simulink model "model_2"  (R2021b)
settings: Solver=FixedStepAuto  StartTime=0.0  StopTime=3  FixedStep=0.00005  RelTol=1e-3
values from neighbouring files (symbols this model uses):
  A = [-6, 0, 0, 0; 0, 8,  0, 0; 0, 0, 2, 5; 0, 0, -5, 2]    [task_1.m]    (also in task_2.m = [0, 7, 0, 0; -7, 0,  0, 0; 0, 0, 0, 1; 0, 0, -1, 0]; task_3.m = [5, -9, -7, 1; -9, 5,  -1, 7; -7, -1, 5, 9; 1, 7, 9, 5])
  B = [0; 1; 9; 2]    [task_1.m]    (also in task_2.m = [0; 0; 0; 0]; task_3.m = [3; 3; 1; 3])
  C = [1, 0, 0, 0; 0, 1, 0, 0; 0, 0, 1, 0; 0, 0, 0, 1]    [task_1.m]    (also in task_2.m = [0, 5, 5, 0]; task_3.m = [2, -2, 2, 2; -2, 4, 2, 4])
  L = inv(Q) * Y    [task_2.m]    (also in task_3.m = inv(Q) * Y1)
  x0 = [1; 1; 1; 1]    [task_2.m]    (also in task_3.m)
  x_0 = [1; 1; 1; 1]    [task_1.m]    (also in task_2.m = [2; 0; 0; -1]; task_3.m = [2; 3; 4; -5])
settings Model: Creator=den  LastModifiedBy=vital

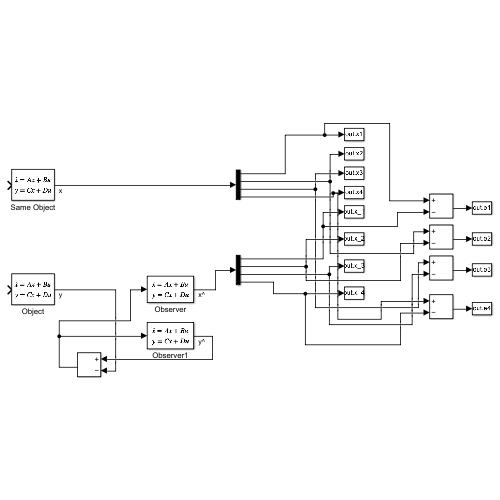
[thumbnail: Simulink's stored preview of the top-level diagram]
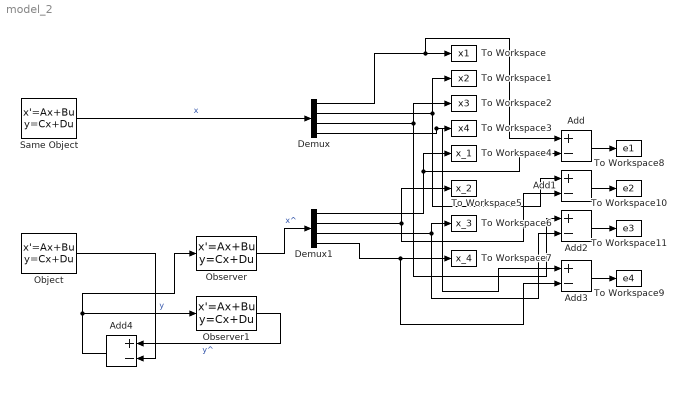
== system model_2 ==
  Add{,1..4} (5 alike) : Sum  Inputs=+-
  Demux : Demux
  Demux1 : Demux
  Object : StateSpace  A=A  B=B  C=C  D=0  InitialCondition=x0
  Observer : StateSpace  A=A  B=L  C=[1,0,0,0; 0,1,0,0; 0,0,1,0; 0,0,0,1]  D=[0;0;0;0]  InitialCondition=x_0  ParameterTunability=Unconstrained
  Observer1 : StateSpace  A=A  B=L  C=C  D=0  InitialCondition=x_0  ParameterTunability=Unconstrained
  Same Object : StateSpace  A=A  B=B  C=[1,0,0,0; 0,1,0,0; 0,0,1,0; 0,0,0,1]  D=[0; 0; 0; 0]  InitialCondition=x0  ParameterTunability=Unconstrained
  To Workspace : ToWorkspace  VariableName=x1  SaveFormat=Timeseries  SampleTime=-1
  To Workspace1 : ToWorkspace  VariableName=x2  SaveFormat=Timeseries  SampleTime=-1
  To Workspace10 : ToWorkspace  VariableName=e2  SaveFormat=Timeseries  SampleTime=-1
  To Workspace11 : ToWorkspace  VariableName=e3  SaveFormat=Timeseries  SampleTime=-1
  To Workspace2 : ToWorkspace  VariableName=x3  SaveFormat=Timeseries  SampleTime=-1
  To Workspace3 : ToWorkspace  VariableName=x4  SaveFormat=Timeseries  SampleTime=-1
  To Workspace4 : ToWorkspace  VariableName=x_1  SaveFormat=Timeseries  SampleTime=-1
  To Workspace5 : ToWorkspace  VariableName=x_2  SaveFormat=Timeseries  SampleTime=-1
  To Workspace6 : ToWorkspace  VariableName=x_3  SaveFormat=Timeseries  SampleTime=-1
  To Workspace7 : ToWorkspace  VariableName=x_4  SaveFormat=Timeseries  SampleTime=-1
  To Workspace8 : ToWorkspace  VariableName=e1  SaveFormat=Timeseries  SampleTime=-1
  To Workspace9 : ToWorkspace  VariableName=e4  SaveFormat=Timeseries  SampleTime=-1
  wires:
  Same Object/1 -> Demux/1  "x"
  Observer/1 -> Demux1/1  "x^"
  Demux/2 -> To Workspace1/1, Add1/1
  Demux/3 -> To Workspace2/1, Add2/1
  Demux/4 -> Add3/1, To Workspace3/1
  Demux1/4 -> Add3/2, To Workspace7/1
  Demux1/3 -> To Workspace6/1, Add2/2
  Demux1/1 -> To Workspace4/1, Add/2
  Demux/1 -> Add/1, To Workspace/1
  Demux1/2 -> To Workspace5/1, Add1/2
  Add/1 -> To Workspace8/1
  Add3/1 -> To Workspace9/1
  Add2/1 -> To Workspace11/1
  Add1/1 -> To Workspace10/1
  Add4/1 -> Observer/1, Observer1/1
  Observer1/1 -> Add4/1  "y^"
  Object/1 -> Add4/2  "y"
